simulink model "uz_mpc_prediction_state_machine"  (R2021a)
settings: Solver=FixedStepDiscrete  StartTime=0.0  StopTime=1/f*3  RelTol=1e-3
values from neighbouring files (symbols this model uses):
  A = 1.0    (= 1)    [uz_6ph_pu_vsd_voltages_init.m]    (also in uz_mpc_6ph_init.m; uz_mpc_6ph_state_machine_init.m)
  f = n_rpm/60.0*p    (= 250)    [uz_6ph_pu_vsd_voltages_init.m]    (also in uz_mpc_6ph_init.m; uz_mpc_6ph_state_machine_init.m)
  Ld_over_LB = Ld/LB    [uz_6ph_pu_vsd_voltages_init.m]    (also in uz_mpc_6ph_init.m; uz_mpc_6ph_state_machine_init.m)
  Lq_over_LB = Lq/LB    [uz_6ph_pu_vsd_voltages_init.m]    (also in uz_mpc_6ph_init.m; uz_mpc_6ph_state_machine_init.m)
  omega_m = n_rpm*pi/30    (= 314.159265359)    [uz_6ph_pu_vsd_voltages_init.m]    (also in uz_mpc_6ph_init.m; uz_mpc_6ph_state_machine_init.m)
  omegaB = nR*2*pi()/60*p    [uz_6ph_pu_vsd_voltages_init.m]    (also in uz_mpc_6ph_init.m; uz_mpc_6ph_state_machine_init.m)
  psi_pm_over_psiB = psi_pm/psiB    [uz_6ph_pu_vsd_voltages_init.m]    (also in uz_mpc_6ph_init.m; uz_mpc_6ph_state_machine_init.m)
  Rs_over_ZB = Rs/ZB    [uz_6ph_pu_vsd_voltages_init.m]    (also in uz_mpc_6ph_init.m; uz_mpc_6ph_state_machine_init.m)
  t_ADC = 1/f_ADC    (= 1e-05)    [uz_6ph_pu_vsd_voltages_init.m]    (also in uz_mpc_6ph_init.m; uz_mpc_6ph_state_machine_init.m; uz_typeconv_init.m)
  t_clock = 1/f_clock    (= 1e-08)    [uz_6ph_pu_vsd_voltages_init.m]    (also in uz_mpc_6ph_init.m; uz_mpc_6ph_state_machine_init.m; uz_typeconv_init.m)
  Ts_times_ZB_over_Ld = Ts*ZB/Ld    [uz_6ph_pu_vsd_voltages_init.m]    (also in uz_mpc_6ph_init.m; uz_mpc_6ph_state_machine_init.m)
  Ts_times_ZB_over_Lq = Ts*ZB/Lq    [uz_6ph_pu_vsd_voltages_init.m]    (also in uz_mpc_6ph_init.m; uz_mpc_6ph_state_machine_init.m)
  Ts_times_ZB_over_Lx = Ts*ZB/Lx    [uz_6ph_pu_vsd_voltages_init.m]    (also in uz_mpc_6ph_init.m; uz_mpc_6ph_state_machine_init.m)
  Ts_times_ZB_over_Ly = Ts*ZB/Ly    [uz_6ph_pu_vsd_voltages_init.m]    (also in uz_mpc_6ph_init.m; uz_mpc_6ph_state_machine_init.m)
  v_dc = 565.0    (= 565)    [uz_6ph_pu_vsd_voltages_init.m]    (also in uz_mpc_6ph_init.m; uz_mpc_6ph_state_machine_init.m)
  VB = sqrt(2/3)*VR    [uz_6ph_pu_vsd_voltages_init.m]    (also in uz_mpc_6ph_init.m; uz_mpc_6ph_state_machine_init.m)
libraries: simulink x9, fl_lib x7, nesl_utility x7, ee_lib x2, hdlsllib x1
(part 1 of 2)
settings Model: DataTypeOverride=Off  Creator=micha  LastModifiedBy=micha
settings SolverCC: AlgebraicLoopSolver=TrustRegion
settings DataIOCC: LimitDataPoints=on  SaveOutput=off  SaveTime=off
settings OptimizationCC: BlockReduction=off  ConditionallyExecuteInputs=off  DefaultParameterBehavior=Inlined  LifeSpan=inf
settings DebuggingCC: AlgebraicLoopMsg=error  SingleTaskRateTransMsg=error  AllowSymbolicDim=off  StrictBusMsg=ErrorOnBusTreatedAsVector  SFUnexpectedBacktrackingDiag=warning  SFNoUnconditionalDefaultTransitionDiag=warning  SFExecutionAtInitializationDiag=none  SFMachineParentedDataDiag=warning  ArithmeticOperatorsInVariantConditions=warning
settings HardwareCC: ProdBitPerPointer=32  ProdBitPerSizeT=32  ProdBitPerPtrDiffT=32  ProdLargestAtomicFloat=None  ProdIntDivRoundTo=Undefined  ProdEndianess=Unspecified  ProdWordSize=32  ProdHWDeviceType=ASIC/FPGA->ASIC/FPGA  ProdEqTarget=off
settings SFSimCC: SimUseLocalCustomCode=off  CustomCodeUndefinedFunction=UseInterfaceOnly
settings RTWCC: RTWUseLocalCustomCode=off
settings CodeAppCC: StateflowObjectComments=on
settings GRTTargetCC: TargetLangStandard=C89/C90 (ANSI)
settings ConfigComp: CovScope=ReferencedModels  CovMetricSettings=dw  CovSaveCumulativeToWorkspaceVar=on  CovSaveSingleToWorkspaceVar=on  CovExternalEMLEnable=off  CovSFcnEnable=off

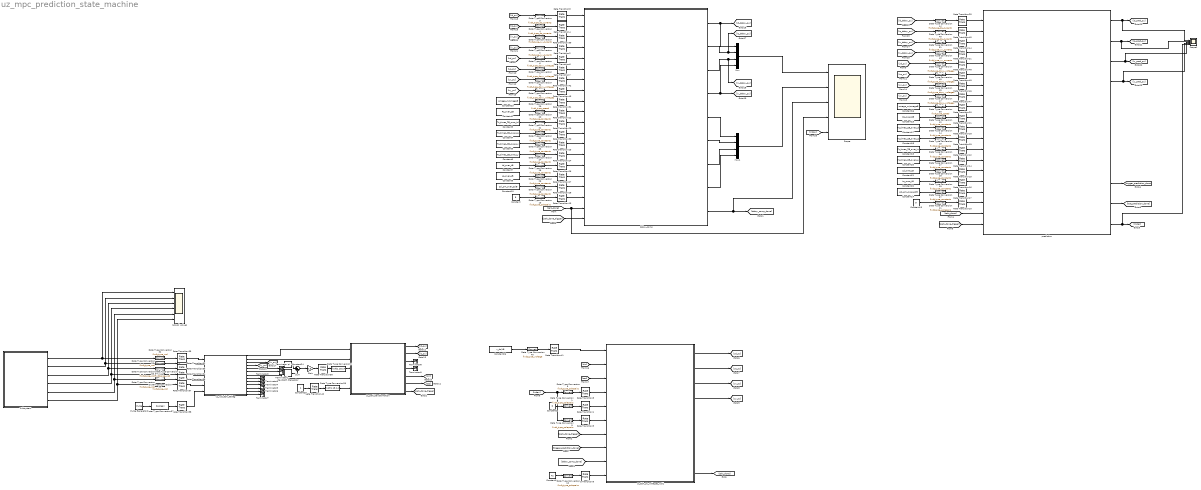
== system uz_mpc_prediction_state_machine ==
  Constant : Constant  Value=5
  Constant1 : Constant  Value=0
  Constant10 : Constant  Value=psi_pm_over_psiB
  Constant12 : Constant  Value=42
  Constant13 : Constant  Value=5
  Constant14 : Constant  Value=psi_pm_over_psiB
  Constant15 : Constant  Value=Rs_over_ZB
  Constant16 : Constant  Value=omega_m/omegaB
  Constant17 : Constant  Value=Ts_times_ZB_over_Ld
  Constant18 : Constant  Value=Ts_times_ZB_over_Lq
  Constant19 : Constant  Value=Ts_times_ZB_over_Lx
  Constant2 : Constant  Value=Rs_over_ZB
  Constant20 : Constant  Value=Ts_times_ZB_over_Ly
  Constant21 : Constant  Value=Ld_over_LB
  Constant22 : Constant  Value=Lq_over_LB
  Constant23 : Constant  Value=omega_m/omegaB
  Constant24 : Constant  Value=2*pi
  Constant25 : Constant
  Constant26 : Constant  Value=v_dc/VB
  Constant3 : Constant  Value=Ts_times_ZB_over_Ld
  Constant4 : Constant  Value=Ts_times_ZB_over_Lq
  Constant5 : Constant  Value=Ts_times_ZB_over_Lx
  Constant6 : Constant  Value=Ts_times_ZB_over_Ly
  Constant7 : Constant  Value=Ld_over_LB
  Constant8 : Constant  Value=Lq_over_LB
  Data Type Conversion{,2,31,43} (4 alike) : DataTypeConversion  OutDataTypeStr=fixdt_type_xy_currents
  Data Type Conversion{1,5,8,10..11,13} (6 alike) : DataTypeConversion  OutDataTypeStr=fixdt_type_polepairs
  Data Type Conversion{12,14..28} (16 alike) : DataTypeConversion  OutDataTypeStr=fixdt_type_constants
  Data Type Conversion29 : DataTypeConversion  OutDataTypeStr=fixdt_type_speed
  Data Type Conversion{3..4,44..45} (4 alike) : DataTypeConversion  OutDataTypeStr=fixdt_type_dq_currents
  Data Type Conversion30 : DataTypeConversion  OutDataTypeStr=fixdt_type_speed
  Data Type Conversion{32..36,38} (6 alike) : DataTypeConversion  OutDataTypeStr=fixdt_type_vsd
  Data Type Conversion37 : DataTypeConversion  OutDataTypeStr=boolean
  Data Type Conversion39 : DataTypeConversion  OutDataTypeStr=fixdt(1,18,14)
  Data Type Conversion40 : DataTypeConversion  OutDataTypeStr=fixdt_type_voltage
  Data Type Conversion{6..7,41..42,46..49} (8 alike) : DataTypeConversion  OutDataTypeStr=fixdt_type_dqxy_voltages
  Data Type Conversion9 : DataTypeConversion  OutDataTypeStr=fixdt(1,18,14)
  Gain : Gain  Gain=0.5
  Mux : Mux
  Mux1 : Mux
  Pulse Generator1 : DiscretePulseGenerator  PulseType=Time based  Period=t_ADC  PulseWidth=5
  Rate Transition{1,5,8..9} (4 alike) : RateTransition  InitialCondition=1  OutPortSampleTime=t_clock
  Rate Transition{2..4,6..7,10..49,58} (46 alike) : RateTransition  OutPortSampleTime=t_clock
  Sawtooth Generator : SignalGenerator  WaveForm=sawtooth  Amplitude=2*pi  Frequency=2*pi*f  Units=rad/sec
  Scope : Scope  NumInputPorts=5
  Scope1 : Scope  NumInputPorts=5
  Subsystem : Subsystem
  Sum : Sum  Inputs=|+-
  Terminator{,1..9} (10 alike) : Terminator
  delay_comp : Subsystem  TreatAsAtomicUnit=on
  natural values : Scope  NumInputPorts=6
  prediction : Subsystem  TreatAsAtomicUnit=on
  uz_6ph_pu_voltages_vsd1 : Subsystem  TreatAsAtomicUnit=on
  uz_park_transformation : Subsystem  TreatAsAtomicUnit=on
  uz_vsd_6ph_30deg : Subsystem  TreatAsAtomicUnit=on
  wires:
  Data Type Conversion24/1 -> Rate Transition24/1
  Constant8/1 -> Data Type Conversion26/1
  Rate Transition22/1 -> delay_comp/10(Rs_over_ZB_AXI)
  Data Type Conversion21/1 -> Rate Transition29/1
  Rate Transition29/1 -> delay_comp/11(Ts_times_ZB_over_Ld_AXI)
  Data Type Conversion26/1 -> Rate Transition27/1
  Constant6/1 -> Data Type Conversion24/1
  Rate Transition30/1 -> delay_comp/12(Ts_times_ZB_over_Lq_AXI)
  Rate Transition27/1 -> delay_comp/16(Lq_over_LB_AXI)
  Constant3/1 -> Data Type Conversion21/1
  Constant2/1 -> Data Type Conversion20/1
  Data Type Conversion25/1 -> Rate Transition26/1
  Data Type Conversion22/1 -> Rate Transition30/1
  Data Type Conversion23/1 -> Rate Transition23/1
  Rate Transition26/1 -> delay_comp/15(Ld_over_LB_AXI)
  Rate Transition24/1 -> delay_comp/14(Ts_times_ZB_over_Ly_AXI)
  Data Type Conversion20/1 -> Rate Transition22/1
  Rate Transition23/1 -> delay_comp/13(Ts_times_ZB_over_Lx_AXI)
  Constant5/1 -> Data Type Conversion23/1
  Constant4/1 -> Data Type Conversion22/1
  Constant7/1 -> Data Type Conversion25/1
  Data Type Conversion29/1 -> Rate Transition31/1
  Constant23/1 -> Data Type Conversion29/1
  Rate Transition31/1 -> delay_comp/9(omega_m_pu)
  Rate Transition2/1 -> delay_comp/4(iy_pu)
  Data Type Conversion3/1 -> Rate Transition3/1
  Rate Transition3/1 -> delay_comp/1(id_pu)
  Data Type Conversion4/1 -> Rate Transition4/1
  Data Type Conversion/1 -> Rate Transition39/1
  Data Type Conversion2/1 -> Rate Transition2/1
  Rate Transition4/1 -> delay_comp/2(iq_pu)
  Rate Transition39/1 -> delay_comp/3(ix_pu)
  Data Type Conversion6/1 -> Rate Transition6/1
  Rate Transition42/1 -> delay_comp/7(vx_pu)
  Data Type Conversion41/1 -> Rate Transition42/1
  Data Type Conversion7/1 -> Rate Transition7/1
  Data Type Conversion42/1 -> Rate Transition43/1
  Rate Transition6/1 -> delay_comp/5(vd_pu)
  Rate Transition7/1 -> delay_comp/6(vq_pu)
  Rate Transition43/1 -> delay_comp/8(vy_pu)
  uz_vsd_6ph_30deg/12(z1_AXI) -> Terminator6/1
  uz_park_transformation/4(y2_AXI) -> Terminator9/1
  uz_vsd_6ph_30deg/8(alpha_AXI) -> Terminator2/1
  uz_vsd_6ph_30deg/13(z2_AXI) -> Terminator7/1
  uz_park_transformation/3(y1_AXI) -> Terminator8/1
  uz_vsd_6ph_30deg/11(y_AXI) -> Terminator5/1
  Subsystem/1(output) -> natural values/1, Data Type Conversion32/1
  Data Type Conversion40/1 -> Rate Transition41/1
  Constant24/1 -> Sum/1
  uz_vsd_6ph_30deg/2(beta) -> uz_park_transformation/2(u2)
  Rate Transition35/1 -> uz_vsd_6ph_30deg/1(a1)
  Pulse Generator1/1 -> Data Type Conversion37/1
  Subsystem/2(output1) -> natural values/2, Data Type Conversion33/1
  uz_vsd_6ph_30deg/7(vsd_done) -> uz_park_transformation/4(trigger)
  Data Type Conversion39/1 -> uz_park_transformation/5(factor_angle_el_AXI)
  uz_vsd_6ph_30deg/1(alpha) -> uz_park_transformation/1(u1)
  Rate Transition41/1 -> uz_6ph_pu_voltages_vsd1/1(v_DC_pu)
  Rate Transition37/1 -> uz_vsd_6ph_30deg/6(c2)
  uz_vsd_6ph_30deg/10(x_AXI) -> Terminator4/1
  uz_vsd_6ph_30deg/6(z2) -> Terminator1/1
  uz_vsd_6ph_30deg/9(beta_AXI) -> Terminator3/1
  Subsystem/5(output4) -> Data Type Conversion36/1, natural values/5
  uz_6ph_pu_voltages_vsd1/9(calc_done) -> [calc_done]  "calc_done"
  Rate Transition33/1 -> uz_vsd_6ph_30deg/3(c1)
  uz_6ph_pu_voltages_vsd1/1(pu_ud) -> [ud_pu]
  Rate Transition38/1 -> Data Type Conversion9/1
  Data Type Conversion38/1 -> Rate Transition37/1
  Subsystem/4(output3) -> Data Type Conversion35/1, natural values/4
  Gain/1 -> Rate Transition38/1
  Rate Transition36/1 -> uz_vsd_6ph_30deg/5(b2)
  Sum/1 -> Gain/1
  Rate Transition58/1 -> uz_vsd_6ph_30deg/7(pu_conv_valid)
  Sawtooth Generator/1 -> Sum/2
  Constant25/1 -> Rate Transition40/1
  Rate Transition40/1 -> Data Type Conversion39/1
  Data Type Conversion34/1 -> Rate Transition33/1
  Subsystem/3(output2) -> Data Type Conversion34/1, natural values/3
  Rate Transition32/1 -> uz_vsd_6ph_30deg/2(b1)
  Subsystem/6(output5) -> natural values/6, Data Type Conversion38/1
  Data Type Conversion33/1 -> Rate Transition32/1
  Data Type Conversion32/1 -> Rate Transition35/1
  uz_vsd_6ph_30deg/5(z1) -> Terminator/1
  Data Type Conversion35/1 -> Rate Transition34/1
  Constant26/1 -> Data Type Conversion40/1
  Data Type Conversion36/1 -> Rate Transition36/1
  Data Type Conversion37/1 -> Rate Transition58/1
  Rate Transition34/1 -> uz_vsd_6ph_30deg/4(a2)
  Constant10/1 -> Data Type Conversion28/1
  Data Type Conversion28/1 -> Rate Transition28/1
  Rate Transition28/1 -> delay_comp/17(psi_pm_over_psiB_AXI)
  Constant/1 -> Data Type Conversion13/1
  Data Type Conversion13/1 -> Rate Transition13/1
  Rate Transition13/1 -> delay_comp/18(polepairs_AXI)
  delay_comp/1(id_delay_pu) -> [id_delay_pu], Mux/1
  delay_comp/2(iq_delay_pu) -> [iq_delay_pu], Mux/2
  delay_comp/3(ix_delay_pu) -> [ix_delay_pu], Mux/3
  delay_comp/4(iy_delay_pu) -> [iy_delay_pu], Mux/4
  Mux/1 -> Scope/1
  delay_comp/6(iq_delay_pu_AXI) -> Mux1/2
  delay_comp/8(iy_delay_pu_AXI) -> Mux1/4
  delay_comp/7(ix_delay_pu_AXI) -> Mux1/3
  delay_comp/5(id_delay_pu_AXI) -> Mux1/1
  Mux1/1 -> Scope/2
  delay_comp/9(calc_done) -> [delay_comp_done], Scope/3
  Rate Transition8/1 -> uz_6ph_pu_voltages_vsd1/4(index)
  Data Type Conversion5/1 -> Rate Transition8/1
  Rate Transition1/1 -> uz_6ph_pu_voltages_vsd1/5(index_select)
  Data Type Conversion1/1 -> Rate Transition1/1
  Constant1/1 -> Data Type Conversion1/1
  Rate Transition5/1 -> uz_6ph_pu_voltages_vsd1/6(index_AXI)
  Data Type Conversion8/1 -> Rate Transition5/1
  [index] -> Data Type Conversion8/1, Data Type Conversion5/1
  Data Type Conversion9/1 -> uz_park_transformation/3(angle_el)
  Data Type Conversion10/1 -> Rate Transition9/1
  Constant12/1 -> Data Type Conversion10/1
  Rate Transition9/1 -> uz_6ph_pu_voltages_vsd1/10(last_opt_index)
  [delay_comp_done] -> uz_6ph_pu_voltages_vsd1/9(trigger_delay_comp_done)
  uz_park_transformation/7(calc_done) -> [park_done_trigger]  "calc_done"
  [park_done_trigger] -> uz_6ph_pu_voltages_vsd1/7(trigger_adc)
  Data Type Conversion11/1 -> Rate Transition10/1
  Constant20/1 -> Data Type Conversion17/1
  Rate Transition10/1 -> prediction/18(polepairs_AXI)
  Constant13/1 -> Data Type Conversion11/1
  Constant14/1 -> Data Type Conversion27/1
  Constant22/1 -> Data Type Conversion19/1
  Data Type Conversion15/1 -> Rate Transition19/1
  Data Type Conversion19/1 -> Rate Transition16/1
  Constant18/1 -> Data Type Conversion15/1
  Rate Transition11/1 -> prediction/10(Rs_over_ZB_AXI)
  Rate Transition18/1 -> prediction/11(Ts_times_ZB_over_Ld_AXI)
  Data Type Conversion12/1 -> Rate Transition11/1
  Data Type Conversion16/1 -> Rate Transition12/1
  Constant16/1 -> Data Type Conversion30/1
  Rate Transition12/1 -> prediction/13(Ts_times_ZB_over_Lx_AXI)
  Rate Transition19/1 -> prediction/12(Ts_times_ZB_over_Lq_AXI)
  Data Type Conversion18/1 -> Rate Transition15/1
  Constant19/1 -> Data Type Conversion16/1
  Constant17/1 -> Data Type Conversion14/1
  Constant21/1 -> Data Type Conversion18/1
  Constant15/1 -> Data Type Conversion12/1
  Data Type Conversion27/1 -> Rate Transition17/1
  Rate Transition17/1 -> prediction/17(psi_pm_over_psiB_AXI)
  Rate Transition16/1 -> prediction/16(Lq_over_LB_AXI)
  Data Type Conversion30/1 -> Rate Transition20/1
  Rate Transition20/1 -> prediction/9(omega_m_pu)
  Rate Transition15/1 -> prediction/15(Ld_over_LB_AXI)
  Data Type Conversion17/1 -> Rate Transition14/1
  Data Type Conversion14/1 -> Rate Transition18/1
  Rate Transition14/1 -> prediction/14(Ts_times_ZB_over_Ly_AXI)
  Data Type Conversion31/1 -> Rate Transition44/1
  Rate Transition48/1 -> prediction/5(vd_pu)
  Data Type Conversion46/1 -> Rate Transition46/1
  Data Type Conversion44/1 -> Rate Transition25/1
  Data Type Conversion49/1 -> Rate Transition49/1
  Rate Transition25/1 -> prediction/1(id_pu)
  Rate Transition46/1 -> prediction/7(vx_pu)
  Data Type Conversion47/1 -> Rate Transition47/1
  Rate Transition47/1 -> prediction/8(vy_pu)
  Data Type Conversion43/1 -> Rate Transition21/1
  Rate Transition21/1 -> prediction/4(iy_pu)
  Data Type Conversion48/1 -> Rate Transition48/1
  Rate Transition44/1 -> prediction/3(ix_pu)
  Rate Transition45/1 -> prediction/2(iq_pu)
  Data Type Conversion45/1 -> Rate Transition45/1
  Rate Transition49/1 -> prediction/6(vq_pu)
  uz_6ph_pu_voltages_vsd1/2(pu_uq) -> [uq_pu]
  prediction/11(index) -> Scope1/5, [index]
  prediction/9(calc_done) -> [trigger_prediction_done]
  [trigger_prediction_done] -> uz_6ph_pu_voltages_vsd1/8(trigger_prediction_done)
  prediction/10(last_prediciton_done) -> [last_prediction_done]
  [calc_done] -> Scope/4, delay_comp/19(trigger_voltages_done)
  [park_done_trigger] -> delay_comp/20(adc_trigger)
  [calc_done] -> prediction/19(trigger_voltages_done)
  [park_done_trigger] -> prediction/20(adc_trigger)
  [ud_pu] -> Data Type Conversion6/1
  [ud_pu] -> Data Type Conversion48/1
  [uq_pu] -> Data Type Conversion7/1
  [uq_pu] -> Data Type Conversion49/1
  uz_6ph_pu_voltages_vsd1/3(pu_ux) -> [ux_pu]
  uz_6ph_pu_voltages_vsd1/4(pu_uy) -> [uy_pu]
  [uy_pu] -> Data Type Conversion42/1
  [ux_pu] -> Data Type Conversion41/1
  [ux_pu] -> Data Type Conversion46/1
  [uy_pu] -> Data Type Conversion47/1
  uz_park_transformation/5(sin) -> [sin]
  uz_park_transformation/6(cos) -> [cos]
  [cos] -> uz_6ph_pu_voltages_vsd1/3(cos_angle)
  [sin] -> uz_6ph_pu_voltages_vsd1/2(sin_angle)
  uz_park_transformation/1(y1) -> [id_pu]
  uz_park_transformation/2(y2) -> [iq_pu]
  [id_pu] -> Data Type Conversion3/1
  [iq_pu] -> Data Type Conversion4/1
  uz_vsd_6ph_30deg/4(y1) -> [iy_pu]
  uz_vsd_6ph_30deg/3(x1) -> [ix_pu]
  [iy_pu] -> Data Type Conversion2/1
  [ix_pu] -> Data Type Conversion/1
  [iy_delay_pu] -> Data Type Conversion43/1
  [ix_delay_pu] -> Data Type Conversion31/1
  [iq_delay_pu] -> Data Type Conversion45/1
  [id_delay_pu] -> Data Type Conversion44/1
  [index] -> Scope/5
  prediction/1(id_pred_pu) -> Scope1/1, [id_pred_pu]
  prediction/2(iq_pred_pu) -> Scope1/2, [iq_pred_pu]
  prediction/3(ix_pred_pu) -> Scope1/3, [ix_pred_pu]
  prediction/4(iy_pred_pu) -> Scope1/4, [iy_pred_pu]

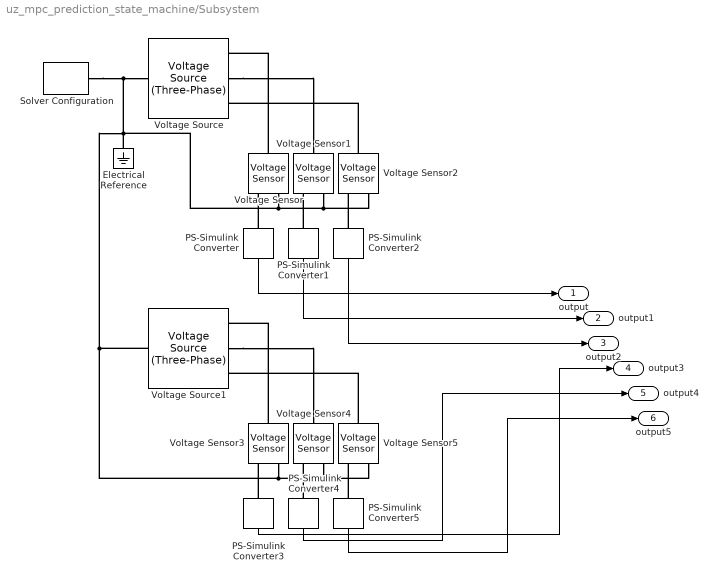
== system uz_mpc_prediction_state_machine/Subsystem ==
  Electrical Reference : fl_lib/Electrical/Electrical Elements/Electrical Reference
  PS-Simulink Converter{,1..5} (6 alike) : nesl_utility/PS-Simulink Converter  PhysicalDomain=network_engine_domain  SubClassName=ps_output  LeftPortType=input  RightPortType=output  PseudoPeriodic=off  Frequencies=[]  Unit=1  AffineConversion=off
  Solver Configuration : nesl_utility/Solver Configuration  PhysicalDomain=network_engine_domain  SubClassName=solver  LeftPortType=input  RightPortType=generic  Tones=[]  Harmonics=[]  SimulateNoise=off  Profile=off  UseLocalSampling=off  EnableSwitchedLinearOptims=on  FrequencyDomain=off  UseCCode=off  RelTol=0.001  AbsTol=1e-06  MinStep=1e-09  ToWorkspace=off  RevertToSquareIcSolve=off  NumHomotopyIterations=100  PhasorMode=off  PhasorModeNumHarmonics=1  DoDC=off  ResidualTolerance=1e-09  UseLocalSolver=on  LocalSolverChoice=NE_BACKWARD_EULER_ADVANCER  LocalSolverSampleTime=1e-6  DoFixedCost=on  MaxNonlinIter=3  MaxModeIter=2  ComputeImpulses=off  ImpulseIterations=2  LinearAlgebra=Sparse  EquationFormulation=NE_TIME_EF  DelaysMemoryBudget=1024  AutomaticFiltering=on  FilteringTimeConstant=0.001  PartitionStorageMethod=AS_NEEDED  PartitionMemoryBudget=1024  PartitionMethod=FAST
  Voltage Sensor{,1..5} (6 alike) : fl_lib/Electrical/Electrical Sensors/Voltage Sensor
  Voltage Source : ee_lib/Sources/Voltage Source (Three-Phase)  vline_rms=A*sqrt(3)/sqrt(2) V  shift=0 deg  freq=f Hz  impedance_option=1  SShortCircuit=1e6 V*A  XR=15  R=0.01 Ohm  L=3.97e-4 H  G_parasitic=0 1/Ohm  harmonic_option=1  harmonic_orders=Harmonic_Orders  harmonic_ratios=Harmonic_Amplitudes  I_specify=off  I_priority=None  I=[ 0 0 0 ] A  I_nominal_specify=off  I_nominal_unit=A  I_nominal_value=1
      settings: SourceProductBaseCode=PS  InternalSimscapePortConfiguration="{\"Bottom\":[],\"Left\":[{\"id\":\"n\",\"label\":\"n\",\"type\":\"foundation.electrical.electrical\"}],\"Right\":[{\"id\":\"a\",\"label\":\"a\",\"type\":\"foundation.electrical.electrical\"},{\"id\":\"b\",\"label\":\"b\",\"type\":\"foundation.electrical.electrical\"},{\"id\":\"c\",\"label\":\"c\",\"type\":\"foundation.electrical.electrical\"}],\"Top\":[]}"
  Voltage Source1 : ee_lib/Sources/Voltage Source (Three-Phase)  vline_rms=A*sqrt(3)/sqrt(2) V  shift=-30 deg  freq=f Hz  impedance_option=1  SShortCircuit=1e6 V*A  XR=15  R=0.01 Ohm  L=3.97e-4 H  G_parasitic=0 1/Ohm  harmonic_option=1  harmonic_orders=Harmonic_Orders  harmonic_ratios=Harmonic_Amplitudes  I_specify=off  I_priority=None  I=[ 0 0 0 ] A  I_nominal_specify=off  I_nominal_unit=A  I_nominal_value=1
      settings: SourceProductBaseCode=PS  InternalSimscapePortConfiguration="{\"Bottom\":[],\"Left\":[{\"id\":\"n\",\"label\":\"n\",\"type\":\"foundation.electrical.electrical\"}],\"Right\":[{\"id\":\"a\",\"label\":\"a\",\"type\":\"foundation.electrical.electrical\"},{\"id\":\"b\",\"label\":\"b\",\"type\":\"foundation.electrical.electrical\"},{\"id\":\"c\",\"label\":\"c\",\"type\":\"foundation.electrical.electrical\"}],\"Top\":[]}"
  output : Outport
  output1 : Outport  Port=2
  output2 : Outport  Port=3
  output3 : Outport  Port=4
  output4 : Outport  Port=5
  output5 : Outport  Port=6
  wires:
  PS-Simulink Converter/1 -> output/1
  PS-Simulink Converter3/1 -> output3/1
  PS-Simulink Converter4/1 -> output4/1
  PS-Simulink Converter1/1 -> output1/1
  PS-Simulink Converter5/1 -> output5/1
  PS-Simulink Converter2/1 -> output2/1
  connections:
  Voltage Sensor5/RConn2 -- Solver Configuration/RConn1 -- Voltage Source/LConn1 -- Voltage Sensor2/RConn2 -- Voltage Sensor1/RConn2 -- Voltage Sensor/RConn2 -- Electrical Reference/LConn1 -- Voltage Source1/LConn1 -- Voltage Sensor3/RConn2 -- Voltage Sensor4/RConn2
  PS-Simulink Converter5/LConn1 -- Voltage Sensor5/RConn1
  PS-Simulink Converter1/LConn1 -- Voltage Sensor1/RConn1
  Voltage Sensor3/LConn1 -- Voltage Source1/RConn1
  PS-Simulink Converter/LConn1 -- Voltage Sensor/RConn1
  Voltage Source1/RConn2 -- Voltage Sensor4/LConn1
  Voltage Sensor5/LConn1 -- Voltage Source1/RConn3
  PS-Simulink Converter4/LConn1 -- Voltage Sensor4/RConn1
  Voltage Sensor2/LConn1 -- Voltage Source/RConn3
  PS-Simulink Converter2/LConn1 -- Voltage Sensor2/RConn1
  PS-Simulink Converter3/LConn1 -- Voltage Sensor3/RConn1
  Voltage Sensor/LConn1 -- Voltage Source/RConn1
  Voltage Source/RConn2 -- Voltage Sensor1/LConn1

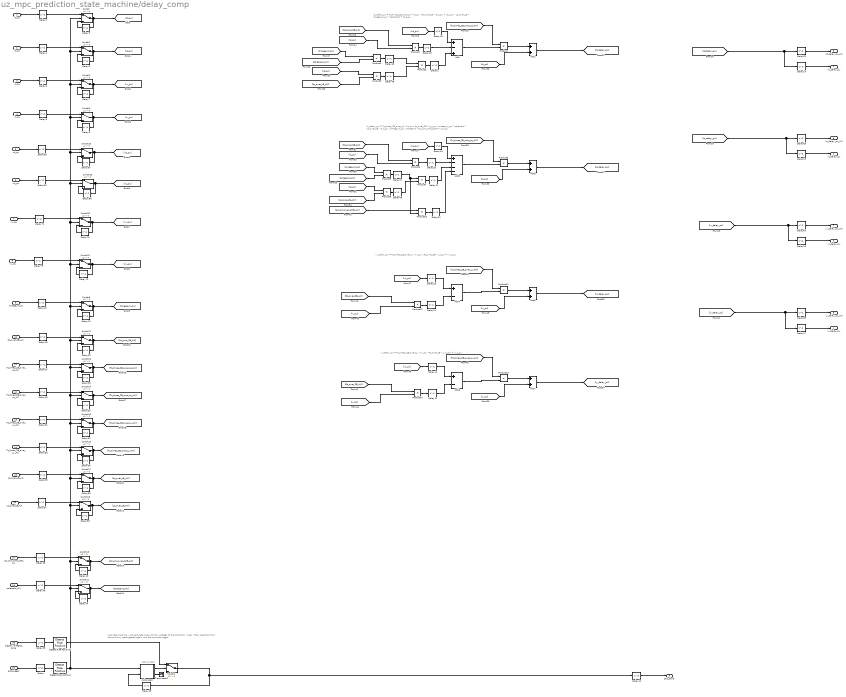
== system uz_mpc_prediction_state_machine/delay_comp ==
  note: mpc state machine - just calculate once with the voltages of the last optim. index. Then reset the S flip flop and only
      | get triggered again with the next adc trigger
  note: iy_delay_pu = Ts_times_ZB_over_Ly *(vy_pu - Rs_over_ZB * iy_k_pu) + iy_k_pu
  note: ix_delay_pu = Ts_times_ZB_over_Lx *(vx_pu - Rs_over_ZB* ix_k_pu) + ix_k_pu
  note: iq_delay_pu = Ts_times_ZB_over_Lq *(vq_pu - Rs_over_ZB * iq_k_pu - omega_m_pu * polepairs * Ld_over_LB * id_k_pu - omega_m_pu * polepairs * psi_pm_over_psiB) + iq_k_pu
  note: id_delay_pu = Ts_times_ZB_over_Ld *(vd_pu - Rs_over_ZB * id_k_pu + iq_k_pu * Lq_over_LB * omega_m_pu * polepairs) + id_k_pu
  note: Q=1 at start
  id_pu : Inport  OutDataTypeStr=fixdt_type_dq_currents
  iq_pu : Inport  Port=2  OutDataTypeStr=fixdt_type_dq_currents
  ix_pu : Inport  Port=3  OutDataTypeStr=fixdt_type_xy_currents
  iy_pu : Inport  Port=4  OutDataTypeStr=fixdt_type_xy_currents
  vd_pu : Inport  Port=5  OutDataTypeStr=fixdt_type_dqxy_voltages
  vq_pu : Inport  Port=6  OutDataTypeStr=fixdt_type_dqxy_voltages
  vx_pu : Inport  Port=7  OutDataTypeStr=fixdt_type_dqxy_voltages
  vy_pu : Inport  Port=8  OutDataTypeStr=fixdt_type_dqxy_voltages
  omega_m_pu : Inport  Port=9  OutDataTypeStr=fixdt_type_speed
  Rs_over_ZB_AXI : Inport  Port=10  OutDataTypeStr=fixdt_type_constants
  Ts_times_ZB_over_Ld_AXI : Inport  Port=11  OutDataTypeStr=fixdt_type_constants
  Ts_times_ZB_over_Lq_AXI : Inport  Port=12  OutDataTypeStr=fixdt_type_constants
  Ts_times_ZB_over_Lx_AXI : Inport  Port=13  OutDataTypeStr=fixdt_type_constants
  Ts_times_ZB_over_Ly_AXI : Inport  Port=14  OutDataTypeStr=fixdt_type_constants
  Ld_over_LB_AXI : Inport  Port=15  OutDataTypeStr=fixdt_type_constants
  Lq_over_LB_AXI : Inport  Port=16  OutDataTypeStr=fixdt_type_constants
  psi_pm_over_psiB_AXI : Inport  Port=17  OutDataTypeStr=fixdt_type_constants
  polepairs_AXI : Inport  Port=18  OutDataTypeStr=fixdt_type_polepairs
  trigger_voltages_done : Inport  Port=19
  adc_trigger : Inport  Port=20
  Add : Sum  Inputs=+-+  AccumDataTypeStr=fixdt(1,27,16)
  Add{1,3,5,7} (4 alike) : Sum  AccumDataTypeStr=fixdt(1,27,24)
  Add2 : Sum  Inputs=+---  AccumDataTypeStr=fixdt(1,27,16)
  Add4 : Sum  Inputs=+-  AccumDataTypeStr=fixdt(1,27,16)
  Add6 : Sum  Inputs=+-  AccumDataTypeStr=fixdt(1,27,16)
  Delay{,2,4,6,8,11..12,14..17,25,27,29,31,33,35,37,39,43,50,59..60,62..65,71,73} (29 alike) : Delay
  Delay{1,3,5,7,9..10,13,18..24,26,28,30,32,34,36,38,40..42,44..49,57..58,70,72} (34 alike) : Delay  DelayLength=1
  Detect Rise Positive : simulink/Logic and Bit Operations/Detect Rise Positive  vinit=0  OutDataTypeStr=boolean
  Detect Rise Positive1 : simulink/Logic and Bit Operations/Detect Rise Positive  vinit=0  OutDataTypeStr=boolean
  Product{,1..2,4..7,9..14} (13 alike) : Product  OutDataTypeStr=fixdt(1,18,15)
  Product3 : Product  OutDataTypeStr=fixdt(1,27,16)
  Product8 : Product  OutDataTypeStr=fixdt(1,27,16)
  Subsystem : Subsystem
  Switch : Switch  Criteria=u2 > Threshold  OutDataTypeStr=fixdt_type_dq_currents
  Switch1 : Switch  Criteria=u2 > Threshold  OutDataTypeStr=fixdt_type_dq_currents
  Switch{12..19} (8 alike) : Switch  Criteria=u2 > Threshold  OutDataTypeStr=fixdt_type_constants
  Switch2 : Switch  Criteria=u2 > Threshold  OutDataTypeStr=fixdt_type_xy_currents
  Switch21 : Switch  Criteria=u2 > Threshold  OutDataTypeStr=fixdt_type_polepairs
  Switch{28..31} (4 alike) : Switch  Criteria=u2 > Threshold  OutDataTypeStr=fixdt_type_dqxy_voltages
  Switch3 : Switch  Criteria=u2 > Threshold  OutDataTypeStr=fixdt_type_xy_currents
  Switch4 : Switch  Criteria=u2 > Threshold
  Switch5 : Switch  Criteria=u2 > Threshold  OutDataTypeStr=fixdt_type_speed
  Terminator2 : Terminator
  id_delay_pu : Outport
  iq_delay_pu : Outport  Port=2
  ix_delay_pu : Outport  Port=3
  iy_delay_pu : Outport  Port=4
  id_delay_pu_AXI : Outport  Port=5
  iq_delay_pu_AXI : Outport  Port=6
  ix_delay_pu_AXI : Outport  Port=7
  iy_delay_pu_AXI : Outport  Port=8
  calc_done : Outport  Port=9
  wires:
  Add5/1 -> [ix_delay_pu]
  Switch12/1 -> [Rs_over_ZB_AXI], Delay26/1
  Add3/1 -> [iq_delay_pu]
  Add1/1 -> [id_delay_pu]
  Add7/1 -> [iy_delay_pu]
  Delay5/1 -> Switch1/3
  Delay25/1 -> Switch12/1
  Delay59/1 -> Switch28/1
  Delay33/1 -> Switch16/1
  vx_pu/1 -> Delay71/1
  vd_pu/1 -> Delay59/1
  Switch15/1 -> [Ts_times_ZB_over_Lx_AXI], Delay32/1
  Ld_over_LB_AXI/1 -> Delay35/1
  Delay2/1 -> Switch/1
  Switch16/1 -> Delay34/1, [Ts_times_ZB_over_Ly_AXI]
  ix_pu/1 -> Delay6/1
  Delay38/1 -> Switch18/3
  Switch17/1 -> Delay36/1, [Ld_over_LB_AXI]
  Delay9/1 -> Switch3/3
  Switch13/1 -> [Ts_times_ZB_over_Ld_AXI], Delay28/1
  Delay/1 -> Detect Rise Positive/1
  Delay34/1 -> Switch16/3
  Delay44/1 -> Switch21/3
  Delay29/1 -> Switch14/1
  Delay8/1 -> Switch3/1
  Switch29/1 -> [vq_pu], Delay58/1
  Switch3/1 -> [iy_pu], Delay9/1
  polepairs_AXI/1 -> Delay43/1
  Delay72/1 -> Switch31/3
  Delay43/1 -> Switch21/1
  Switch14/1 -> [Ts_times_ZB_over_Lq_AXI], Delay30/1
  Delay28/1 -> Switch13/3
  psi_pm_over_psiB_AXI/1 -> Delay39/1
  Delay58/1 -> Switch29/3
  id_pu/1 -> Delay2/1
  Switch21/1 -> [polepairs_AXI], Delay44/1
  Switch/1 -> [id_pu], Delay3/1
  Delay35/1 -> Switch17/1
  Delay31/1 -> Switch15/1
  Switch28/1 -> [vd_pu], Delay57/1
  Ts_times_ZB_over_Ly_AXI/1 -> Delay33/1
  Delay7/1 -> Switch2/3
  Delay37/1 -> Switch18/1
  Delay4/1 -> Switch1/1
  Switch2/1 -> [ix_pu], Delay7/1
  Delay12/1 -> Switch5/1
  Delay73/1 -> Switch31/1
  Switch31/1 -> Delay72/1, [vy_pu]
  omega_m_pu/1 -> Delay12/1
  Delay6/1 -> Switch2/1
  Delay27/1 -> Switch13/1
  vq_pu/1 -> Delay60/1
  Switch5/1 -> [omega_m_pu], Delay13/1
  Lq_over_LB_AXI/1 -> Delay37/1
  iq_pu/1 -> Delay4/1
  iy_pu/1 -> Delay8/1
  vy_pu/1 -> Delay73/1
  Delay70/1 -> Switch30/3
  Delay60/1 -> Switch29/1
  Switch30/1 -> Delay70/1, [vx_pu]
  Ts_times_ZB_over_Lq_AXI/1 -> Delay29/1
  Delay3/1 -> Switch/3
  Switch18/1 -> Delay38/1, [Lq_over_LB_AXI]
  Delay26/1 -> Switch12/3
  Switch19/1 -> [psi_pm_over_psiB_AXI], Delay40/1
  Ts_times_ZB_over_Lx_AXI/1 -> Delay31/1
  Delay71/1 -> Switch30/1
  Switch1/1 -> [iq_pu], Delay5/1
  Ts_times_ZB_over_Ld_AXI/1 -> Delay27/1
  Delay57/1 -> Switch28/3
  Rs_over_ZB_AXI/1 -> Delay25/1
  Delay39/1 -> Switch19/1
  adc_trigger/1 -> Delay/1
  Delay40/1 -> Switch19/3
  Delay13/1 -> Switch5/3
  Delay32/1 -> Switch15/3
  Delay36/1 -> Switch17/3
  Delay30/1 -> Switch14/3
  Delay11/1 -> calc_done/1
  [iy_delay_pu] -> Delay17/1, Delay65/1
  [iq_delay_pu] -> Delay15/1, Delay63/1
  [id_delay_pu] -> Delay14/1, Delay62/1
  Delay63/1 -> iq_delay_pu_AXI/1
  Delay65/1 -> iy_delay_pu_AXI/1
  Delay64/1 -> ix_delay_pu_AXI/1
  [ix_delay_pu] -> Delay16/1, Delay64/1
  Delay62/1 -> id_delay_pu_AXI/1
  Delay15/1 -> iq_delay_pu/1
  Delay14/1 -> id_delay_pu/1
  Delay16/1 -> ix_delay_pu/1
  Delay17/1 -> iy_delay_pu/1
  Add/1 -> Product/2
  [Ts_times_ZB_over_Ld_AXI] -> Product/1  "Ts_times_ZB_over_Ld"
  Product/1 -> Add1/1
  [id_pu] -> Add1/2  "id_k_pu"
  [Rs_over_ZB_AXI] -> Product1/1  "Rs_over_ZB"
  [id_pu] -> Product1/2  "id_k_pu"
  [iq_pu] -> Product3/1  "iq_k_pu"
  [Lq_over_LB_AXI] -> Product3/2  "Lq_over_LB"
  [omega_m_pu] -> Product4/1  "omega_m_pu"
  [polepairs_AXI] -> Product4/2  "polepairs"
  [Ts_times_ZB_over_Lq_AXI] -> Product5/1  "Ts_times_ZB_over_Lq"
  [iq_pu] -> Product6/2  "iq_k_pu"
  [Rs_over_ZB_AXI] -> Product6/1  "Rs_over_ZB"
  Add2/1 -> Product5/2
  [omega_m_pu] -> Product9/1  "omega_m_pu"
  [iq_pu] -> Add3/2  "iq_k_pu"
  [id_pu] -> Product8/1  "id_k_pu"
  [Ld_over_LB_AXI] -> Product8/2  "Ld_over_LB"
  [polepairs_AXI] -> Product9/2  "polepairs"
  Product5/1 -> Add3/1
  [psi_pm_over_psiB_AXI] -> Product10/1
  [Ts_times_ZB_over_Lx_AXI] -> Product11/1  "Ts_times_ZB_over_Lx"
  [ix_pu] -> Product12/2  "ix_k_pu"
  [Rs_over_ZB_AXI] -> Product12/1  "Rs_over_ZB"
  Add4/1 -> Product11/2
  [ix_pu] -> Add5/2  "ix_k_pu"
  Product11/1 -> Add5/1
  [Rs_over_ZB_AXI] -> Product14/1  "Rs_over_ZB"
  Add6/1 -> Product13/2
  [iy_pu] -> Add7/2  "iy_k_pu"
  [iy_pu] -> Product14/2  "iy_k_pu"
  [Ts_times_ZB_over_Ly_AXI] -> Product13/1  "Ts_times_ZB_over_Ly"
  Product13/1 -> Add7/1
  Product2/1 -> Delay1/1
  Product1/1 -> Delay10/1
  Delay10/1 -> Add/2
  Delay1/1 -> Add/3
  [vd_pu] -> Delay18/1  "vd_pu"
  Delay18/1 -> Add/1
  [vq_pu] -> Delay19/1  "vq_pu"
  Product7/1 -> Delay21/1
  Product10/1 -> Delay22/1
  Delay22/1 -> Add2/4
  Delay21/1 -> Add2/3
  Delay20/1 -> Add2/2
  Delay19/1 -> Add2/1
  Product6/1 -> Delay20/1
  [vx_pu] -> Delay23/1  "vx_pu"
  Delay23/1 -> Add4/1
  Product12/1 -> Delay24/1
  Delay24/1 -> Add4/2
  [vy_pu] -> Delay41/1  "vy_pu"
  Product14/1 -> Delay42/1
  Delay42/1 -> Add6/2
  Delay41/1 -> Add6/1
  Product4/1 -> Delay45/1
  Product3/1 -> Delay46/1
  Delay46/1 -> Product2/2
  Delay45/1 -> Product2/1
  Product9/1 -> Delay47/1
  Delay47/1 -> Product10/2, Product7/1
  Product8/1 -> Delay48/1
  Delay48/1 -> Product7/2
  Delay49/1 -> Subsystem/2(Reset)
  Switch4/1 -> Delay49/1, Delay11/1  "delay_comp_done"
  Detect Rise Positive1/1 -> Switch4/1  "delay_comp done"
  Subsystem/1(Q) -> Switch4/2  "Q"
  Subsystem/2(!Q) -> Terminator2/1
  trigger_voltages_done/1 -> Delay50/1
  Delay50/1 -> Detect Rise Positive1/1
  Detect Rise Positive/1 -> Subsystem/1(Set), Switch21/2, Switch19/2, Switch18/2, Switch17/2, Switch16/2, Switch15/2, Switch14/2, Switch13/2, Switch12/2, Switch5/2, Switch31/2, Switch30/2, Switch29/2, Switch28/2, Switch3/2, Switch2/2, Switch1/2, Switch/2

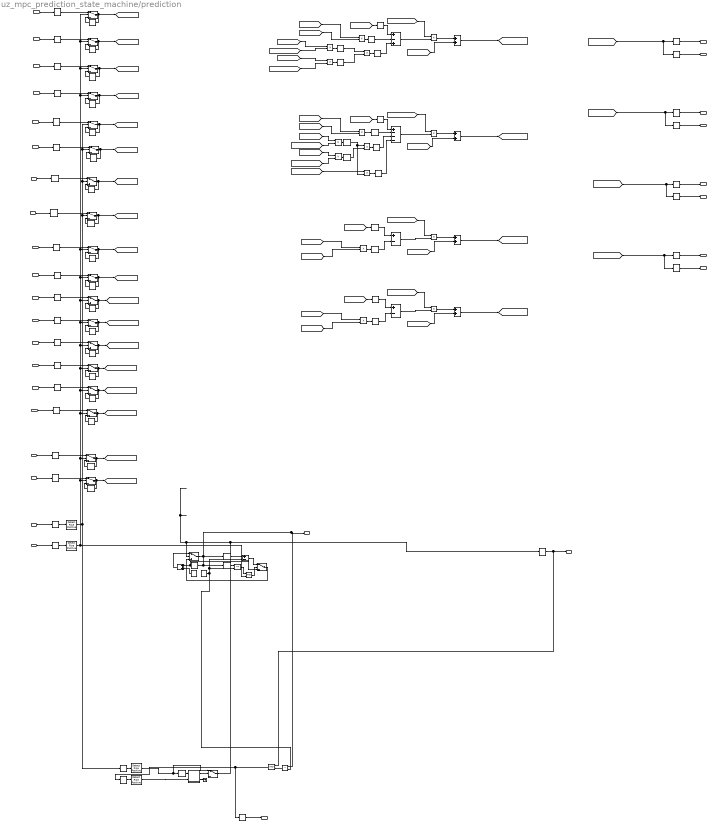
== system uz_mpc_prediction_state_machine/prediction ==
  note: voltages are triggered from voltage calculation ip every iteration
  note: iy_delay_pu = Ts_times_ZB_over_Ly *(vy_pu - Rs_over_ZB * iy_k_pu) + iy_k_pu
  note: ix_delay_pu = Ts_times_ZB_over_Lx *(vx_pu - Rs_over_ZB* ix_k_pu) + ix_k_pu
  note: iq_delay_pu = Ts_times_ZB_over_Lq *(vq_pu - Rs_over_ZB * iq_k_pu - omega_m_pu * polepairs * Ld_over_LB * id_k_pu - omega_m_pu * polepairs * psi_pm_over_psiB) + iq_k_pu
  note: id_delay_pu = Ts_times_ZB_over_Ld *(vd_pu - Rs_over_ZB * id_k_pu + iq_k_pu * Lq_over_LB * omega_m_pu * polepairs) + id_k_pu
  note: counter with adjustable reset
  note: mpc state machine
  id_pu : Inport  OutDataTypeStr=fixdt_type_dq_currents
  iq_pu : Inport  Port=2  OutDataTypeStr=fixdt_type_dq_currents
  ix_pu : Inport  Port=3  OutDataTypeStr=fixdt_type_xy_currents
  iy_pu : Inport  Port=4  OutDataTypeStr=fixdt_type_xy_currents
  vd_pu : Inport  Port=5  OutDataTypeStr=fixdt_type_dqxy_voltages
  vq_pu : Inport  Port=6  OutDataTypeStr=fixdt_type_dqxy_voltages
  vx_pu : Inport  Port=7  OutDataTypeStr=fixdt_type_dqxy_voltages
  vy_pu : Inport  Port=8  OutDataTypeStr=fixdt_type_dqxy_voltages
  omega_m_pu : Inport  Port=9  OutDataTypeStr=fixdt_type_speed
  Rs_over_ZB_AXI : Inport  Port=10  OutDataTypeStr=fixdt_type_constants
  Ts_times_ZB_over_Ld_AXI : Inport  Port=11  OutDataTypeStr=fixdt_type_constants
  Ts_times_ZB_over_Lq_AXI : Inport  Port=12  OutDataTypeStr=fixdt_type_constants
  Ts_times_ZB_over_Lx_AXI : Inport  Port=13  OutDataTypeStr=fixdt_type_constants
  Ts_times_ZB_over_Ly_AXI : Inport  Port=14  OutDataTypeStr=fixdt_type_constants
  Ld_over_LB_AXI : Inport  Port=15  OutDataTypeStr=fixdt_type_constants
  Lq_over_LB_AXI : Inport  Port=16  OutDataTypeStr=fixdt_type_constants
  psi_pm_over_psiB_AXI : Inport  Port=17  OutDataTypeStr=fixdt_type_constants
  polepairs_AXI : Inport  Port=18  OutDataTypeStr=fixdt_type_polepairs
  trigger_voltages_done : Inport  Port=19
  adc_trigger : Inport  Port=20
  Add : Sum  Inputs=+-+  AccumDataTypeStr=fixdt(1,27,16)
  Add{1,3,5,7} (4 alike) : Sum  AccumDataTypeStr=fixdt(1,27,24)
  Add2 : Sum  Inputs=+---  AccumDataTypeStr=fixdt(1,27,16)
  Add4 : Sum  Inputs=+-  AccumDataTypeStr=fixdt(1,27,16)
  Add6 : Sum  Inputs=+-  AccumDataTypeStr=fixdt(1,27,16)
  Add8 : Sum  AccumDataTypeStr=uint32
  Add9 : Sum  Inputs=+-  AccumDataTypeStr=uint32
  Constant : Constant  OutDataTypeStr=uint32  SampleTime=-1
  Constant1 : Constant  Value=63  OutDataTypeStr=uint32  SampleTime=-1
  Delay{,2,4,6,8,11..12,14..17,25,27,29,31,33,35,37,39,43,50,59..60,62..65,71,73} (29 alike) : Delay
  Delay{1,3,5,7,9..10,13,18..24,26,28,30,32,34,36,38,40..42,44..48,53..58,70,72} (37 alike) : Delay  DelayLength=1
  Delay49 : Delay  DelayLength=1  InitialCondition=1
  Delay51 : Delay  DelayLength=1  InitialCondition=1
  Delay52 : Delay  DelayLength=1  InitialCondition=1
  Detect Rise Positive{,1..3} (4 alike) : simulink/Logic and Bit Operations/Detect Rise Positive  vinit=0  OutDataTypeStr=boolean
  Logical Operator : Logic  AllPortsSameDT=off  OutDataTypeStr=boolean
  Logical Operator1 : Logic  AllPortsSameDT=off  OutDataTypeStr=boolean
  Product{,1..2,4..7,9..14} (13 alike) : Product  OutDataTypeStr=fixdt(1,18,15)
  Product3 : Product  OutDataTypeStr=fixdt(1,27,16)
  Product8 : Product  OutDataTypeStr=fixdt(1,27,16)
  Relational Operator : RelationalOperator  OutDataTypeStr=boolean  RndMeth=Simplest
  Relational Operator1 : RelationalOperator  Operator=>  OutDataTypeStr=boolean  RndMeth=Simplest
  Subsystem : Subsystem
  Switch : Switch  Criteria=u2 > Threshold  OutDataTypeStr=fixdt_type_dq_currents
  Switch1 : Switch  Criteria=u2 > Threshold  OutDataTypeStr=fixdt_type_dq_currents
  Switch{12..19} (8 alike) : Switch  Criteria=u2 > Threshold  OutDataTypeStr=fixdt_type_constants
  Switch2 : Switch  Criteria=u2 > Threshold  OutDataTypeStr=fixdt_type_xy_currents
  Switch21 : Switch  Criteria=u2 > Threshold  OutDataTypeStr=fixdt_type_polepairs
  Switch{28..31} (4 alike) : Switch  Criteria=u2 > Threshold  OutDataTypeStr=fixdt_type_dqxy_voltages
  Switch3 : Switch  Criteria=u2 > Threshold  OutDataTypeStr=fixdt_type_xy_currents
  Switch4 : Switch  Criteria=u2 > Threshold
  Switch5 : Switch  Criteria=u2 > Threshold  OutDataTypeStr=fixdt_type_speed
  Switch6 : Switch  Criteria=u2 > Threshold
  Switch7 : Switch  Criteria=u2 > Threshold
  Terminator1 : Terminator
  id_pred_pu : Outport
  iq_pred_pu : Outport  Port=2
  ix_pred_pu : Outport  Port=3
  iy_pred_pu : Outport  Port=4
  id_pred_pu_AXI : Outport  Port=5
  iq_pred_pu_AXI : Outport  Port=6
  ix_pred_pu_AXI : Outport  Port=7
  iy_pred_pu_AXI : Outport  Port=8
  calc_done : Outport  Port=9
  last_prediciton_done : Outport  Port=10  VectorParamsAs1DForOutWhenUnconnected=off
  index : Outport  Port=11  VectorParamsAs1DForOutWhenUnconnected=off
  wires:
  Add5/1 -> [ix_delay_pu]
  Switch12/1 -> [Rs_over_ZB_AXI], Delay26/1
  Add3/1 -> [iq_delay_pu]
  Add1/1 -> [id_delay_pu]
  Add7/1 -> [iy_delay_pu]
  Delay5/1 -> Switch1/3
  Delay25/1 -> Switch12/1
  Delay59/1 -> Switch28/1
  Delay33/1 -> Switch16/1
  vx_pu/1 -> Delay71/1
  vd_pu/1 -> Delay59/1
  Switch15/1 -> [Ts_times_ZB_over_Lx_AXI], Delay32/1
  Ld_over_LB_AXI/1 -> Delay35/1
  Delay2/1 -> Switch/1
  Switch16/1 -> Delay34/1, [Ts_times_ZB_over_Ly_AXI]
  ix_pu/1 -> Delay6/1
  Delay38/1 -> Switch18/3
  Switch17/1 -> Delay36/1, [Ld_over_LB_AXI]
  Delay9/1 -> Switch3/3
  Switch13/1 -> [Ts_times_ZB_over_Ld_AXI], Delay28/1
  Delay/1 -> Detect Rise Positive/1
  Delay34/1 -> Switch16/3
  Delay44/1 -> Switch21/3
  Delay29/1 -> Switch14/1
  Delay8/1 -> Switch3/1
  Switch29/1 -> [vq_pu], Delay58/1
  Switch3/1 -> [iy_pu], Delay9/1
  polepairs_AXI/1 -> Delay43/1
  Delay72/1 -> Switch31/3
  Delay43/1 -> Switch21/1
  Switch14/1 -> [Ts_times_ZB_over_Lq_AXI], Delay30/1
  Delay28/1 -> Switch13/3
  psi_pm_over_psiB_AXI/1 -> Delay39/1
  Delay58/1 -> Switch29/3
  id_pu/1 -> Delay2/1
  Switch21/1 -> [polepairs_AXI], Delay44/1
  Switch/1 -> [id_pu], Delay3/1
  Delay35/1 -> Switch17/1
  Delay31/1 -> Switch15/1
  Switch28/1 -> [vd_pu], Delay57/1
  Ts_times_ZB_over_Ly_AXI/1 -> Delay33/1
  Delay7/1 -> Switch2/3
  Delay37/1 -> Switch18/1
  Delay4/1 -> Switch1/1
  Switch2/1 -> [ix_pu], Delay7/1
  Delay12/1 -> Switch5/1
  Delay73/1 -> Switch31/1
  Switch31/1 -> Delay72/1, [vy_pu]
  omega_m_pu/1 -> Delay12/1
  Delay6/1 -> Switch2/1
  Delay27/1 -> Switch13/1
  vq_pu/1 -> Delay60/1
  Switch5/1 -> [omega_m_pu], Delay13/1
  Lq_over_LB_AXI/1 -> Delay37/1
  iq_pu/1 -> Delay4/1
  iy_pu/1 -> Delay8/1
  vy_pu/1 -> Delay73/1
  Delay70/1 -> Switch30/3
  Delay60/1 -> Switch29/1
  Switch30/1 -> Delay70/1, [vx_pu]
  Ts_times_ZB_over_Lq_AXI/1 -> Delay29/1
  Delay3/1 -> Switch/3
  Switch18/1 -> Delay38/1, [Lq_over_LB_AXI]
  Delay26/1 -> Switch12/3
  Switch19/1 -> [psi_pm_over_psiB_AXI], Delay40/1
  Ts_times_ZB_over_Lx_AXI/1 -> Delay31/1
  Delay71/1 -> Switch30/1
  Switch1/1 -> [iq_pu], Delay5/1
  Ts_times_ZB_over_Ld_AXI/1 -> Delay27/1
  Delay57/1 -> Switch28/3
  Rs_over_ZB_AXI/1 -> Delay25/1
  Delay39/1 -> Switch19/1
  adc_trigger/1 -> Delay/1
  Delay40/1 -> Switch19/3
  Delay13/1 -> Switch5/3
  Delay32/1 -> Switch15/3
  Delay36/1 -> Switch17/3
  Delay30/1 -> Switch14/3
  Delay11/1 -> Logical Operator1/1, calc_done/1
  [iy_delay_pu] -> Delay17/1, Delay65/1
  [iq_delay_pu] -> Delay15/1, Delay63/1
  [id_delay_pu] -> Delay14/1, Delay62/1
  Delay63/1 -> iq_pred_pu_AXI/1
  Delay65/1 -> iy_pred_pu_AXI/1
  Delay64/1 -> ix_pred_pu_AXI/1
  [ix_delay_pu] -> Delay16/1, Delay64/1
  Delay62/1 -> id_pred_pu_AXI/1
  Delay15/1 -> iq_pred_pu/1
  Delay14/1 -> id_pred_pu/1
  Delay16/1 -> ix_pred_pu/1
  Delay17/1 -> iy_pred_pu/1
  Add/1 -> Product/2
  [Ts_times_ZB_over_Ld_AXI] -> Product/1  "Ts_times_ZB_over_Ld"
  Product/1 -> Add1/1
  [id_pu] -> Add1/2  "id_k_pu"
  [Rs_over_ZB_AXI] -> Product1/1  "Rs_over_ZB"
  [id_pu] -> Product1/2  "id_k_pu"
  [iq_pu] -> Product3/1  "iq_k_pu"
  [Lq_over_LB_AXI] -> Product3/2  "Lq_over_LB"
  [omega_m_pu] -> Product4/1  "omega_m_pu"
  [polepairs_AXI] -> Product4/2  "polepairs"
  [Ts_times_ZB_over_Lq_AXI] -> Product5/1  "Ts_times_ZB_over_Lq"
  [iq_pu] -> Product6/2  "iq_k_pu"
  [Rs_over_ZB_AXI] -> Product6/1  "Rs_over_ZB"
  Add2/1 -> Product5/2
  [omega_m_pu] -> Product9/1  "omega_m_pu"
  [iq_pu] -> Add3/2  "iq_k_pu"
  [id_pu] -> Product8/1  "id_k_pu"
  [Ld_over_LB_AXI] -> Product8/2  "Ld_over_LB"
  [polepairs_AXI] -> Product9/2  "polepairs"
  Product5/1 -> Add3/1
  [psi_pm_over_psiB_AXI] -> Product10/1
  [Ts_times_ZB_over_Lx_AXI] -> Product11/1  "Ts_times_ZB_over_Lx"
  [ix_pu] -> Product12/2  "ix_k_pu"
  [Rs_over_ZB_AXI] -> Product12/1  "Rs_over_ZB"
  Add4/1 -> Product11/2
  [ix_pu] -> Add5/2  "ix_k_pu"
  Product11/1 -> Add5/1
  [Rs_over_ZB_AXI] -> Product14/1  "Rs_over_ZB"
  Add6/1 -> Product13/2
  [iy_pu] -> Add7/2  "iy_k_pu"
  [iy_pu] -> Product14/2  "iy_k_pu"
  [Ts_times_ZB_over_Ly_AXI] -> Product13/1  "Ts_times_ZB_over_Ly"
  Product13/1 -> Add7/1
  Product2/1 -> Delay1/1
  Product1/1 -> Delay10/1
  Delay10/1 -> Add/2
  Delay1/1 -> Add/3
  [vd_pu] -> Delay18/1  "vd_pu"
  Delay18/1 -> Add/1
  [vq_pu] -> Delay19/1  "vq_pu"
  Product7/1 -> Delay21/1
  Product10/1 -> Delay22/1
  Delay22/1 -> Add2/4
  Delay21/1 -> Add2/3
  Delay20/1 -> Add2/2
  Delay19/1 -> Add2/1
  Product6/1 -> Delay20/1
  [vx_pu] -> Delay23/1  "vx_pu"
  Delay23/1 -> Add4/1
  Product12/1 -> Delay24/1
  Delay24/1 -> Add4/2
  [vy_pu] -> Delay41/1  "vy_pu"
  Product14/1 -> Delay42/1
  Delay42/1 -> Add6/2
  Delay41/1 -> Add6/1
  Product4/1 -> Delay45/1
  Product3/1 -> Delay46/1
  Delay46/1 -> Product2/2
  Delay45/1 -> Product2/1
  Product9/1 -> Delay47/1
  Delay47/1 -> Product10/2, Product7/1
  Product8/1 -> Delay48/1
  Delay48/1 -> Product7/2
  Detect Rise Positive1/1 -> Delay53/1, Switch31/2, Switch30/2, Switch29/2, Switch28/2  "delay_comp done"
  trigger_voltages_done/1 -> Delay50/1
  Delay50/1 -> Detect Rise Positive1/1
  Add8/1 -> Switch4/1
  Relational Operator/1 -> Logical Operator/1
  Delay52/1 -> Add9/1
  Switch7/1 -> Switch4/2, Delay11/1  "trigger_predict"
  Detect Rise Positive/1 -> Switch21/2, Switch19/2, Switch18/2, Switch17/2, Switch16/2, Switch15/2, Switch14/2, Switch13/2, Switch12/2, Switch5/2, Switch3/2, Switch2/2, Switch1/2, Switch/2, Logical Operator/2
  Delay49/1 -> Switch6/3, Add8/1
  Add9/1 -> Switch6/1
  Constant/1 -> Add8/2
  Logical Operator/1 -> Switch6/2
  Delay51/1 -> Relational Operator/1
  Switch6/1 -> Switch4/3
  Switch4/1 -> Delay52/1, index/1, Relational Operator1/1, Delay49/1, Delay51/1  "predict done"
  Delay56/1 -> last_prediciton_done/1  "predict done"
  Detect Rise Positive3/1 -> Subsystem/2(Reset)
  Relational Operator1/1 -> Logical Operator1/2
  Delay54/1 -> Detect Rise Positive3/1
  Delay55/1 -> Subsystem/1(Set)
  Logical Operator1/1 -> Delay56/1, Delay54/1
  Subsystem/2(!Q) -> Terminator1/1
  Detect Rise Positive2/1 -> Switch7/1, Delay55/1
  Subsystem/1(Q) -> Switch7/2  "Q"
  Constant1/1 -> Relational Operator1/2, Add9/2, Relational Operator/2
  Delay53/1 -> Detect Rise Positive2/1

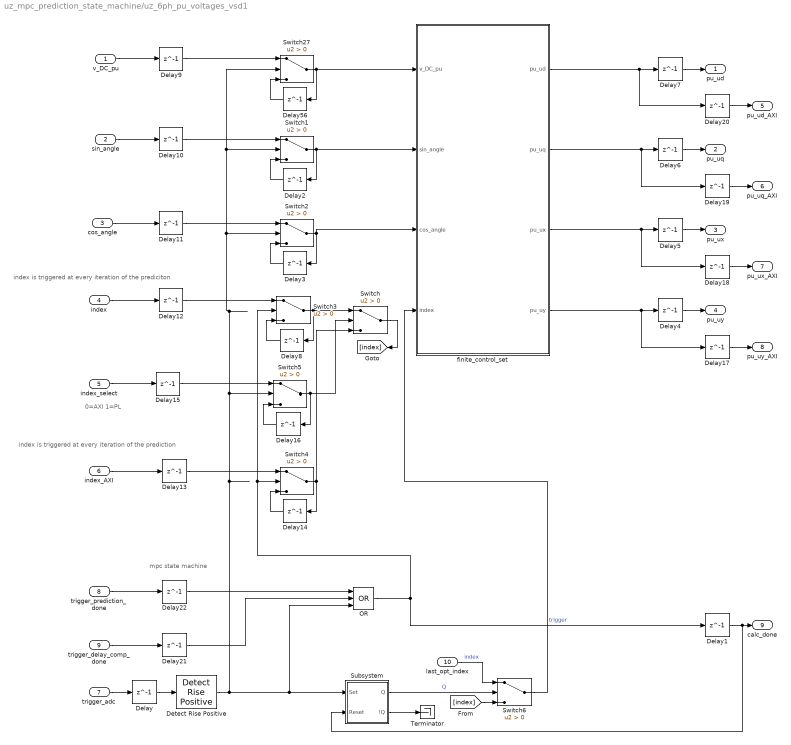
== system uz_mpc_prediction_state_machine/uz_6ph_pu_voltages_vsd1 ==
  note: index is triggered at every iteration of the prediction
  note: index is triggered at every iteration of the prediciton
  note: 0=AXI 1=PL
  note: mpc state machine
  v_DC_pu : Inport  OutDataTypeStr=fixdt_type_constants
  sin_angle : Inport  Port=2  OutDataTypeStr=fixdt_type_sin_cos
  cos_angle : Inport  Port=3  OutDataTypeStr=fixdt_type_sin_cos
  index : Inport  Port=4
  index_select : Inport  Port=5
  index_AXI : Inport  Port=6
  trigger_adc : Inport  Port=7
  trigger_prediction_done : Inport  Port=8
  trigger_delay_comp_done : Inport  Port=9
  last_opt_index : Inport  Port=10
  Delay{,1..7,9..13,15,17..22,56} (21 alike) : Delay  DelayLength=1
  Delay14 : Delay  DelayLength=1  InitialCondition=1
  Delay16 : Delay  DelayLength=1  InitialCondition=1
  Delay8 : Delay  DelayLength=1  InitialCondition=1
  Detect Rise Positive : simulink/Logic and Bit Operations/Detect Rise Positive  vinit=0  OutDataTypeStr=boolean
  OR : Logic  Operator=OR  Inputs=3  IconShape=distinctive  AllPortsSameDT=off  OutDataTypeStr=boolean
  Subsystem : Subsystem
  Switch : Switch  Criteria=u2 > Threshold
  Switch1 : Switch  Criteria=u2 > Threshold  OutDataTypeStr=fixdt_type_sin_cos
  Switch2 : Switch  Criteria=u2 > Threshold  OutDataTypeStr=fixdt_type_sin_cos
  Switch27 : Switch  Criteria=u2 > Threshold  OutDataTypeStr=fixdt_type_constants
  Switch3 : Switch  Criteria=u2 > Threshold  OutDataTypeStr=fixdt_type_polepairs
  Switch4 : Switch  Criteria=u2 > Threshold  OutDataTypeStr=fixdt_type_polepairs
  Switch5 : Switch  Criteria=u2 > Threshold  OutDataTypeStr=fixdt_type_polepairs
  Switch6 : Switch  Criteria=u2 > Threshold
  Terminator : Terminator
  finite_control_set : MATLAB Function  TreatAsAtomicUnit=on
  pu_ud : Outport
  pu_uq : Outport  Port=2
  pu_ux : Outport  Port=3
  pu_uy : Outport  Port=4
  pu_ud_AXI : Outport  Port=5
  pu_uq_AXI : Outport  Port=6
  pu_ux_AXI : Outport  Port=7
  pu_uy_AXI : Outport  Port=8
  calc_done : Outport  Port=9
  wires:
  finite_control_set/1(pu_ud) -> Delay20/1, Delay7/1
  finite_control_set/2(pu_uq) -> Delay19/1, Delay6/1
  finite_control_set/3(pu_ux) -> Delay18/1, Delay5/1
  finite_control_set/4(pu_uy) -> Delay17/1, Delay4/1
  trigger_adc/1 -> Delay/1
  Delay/1 -> Detect Rise Positive/1
  Delay56/1 -> Switch27/3
  v_DC_pu/1 -> Delay9/1
  Switch27/1 -> Delay56/1, finite_control_set/1(v_DC_pu)
  sin_angle/1 -> Delay10/1
  Delay2/1 -> Switch1/3
  Switch1/1 -> finite_control_set/2(sin_angle), Delay2/1
  cos_angle/1 -> Delay11/1
  Delay3/1 -> Switch2/3
  Switch2/1 -> finite_control_set/3(cos_angle), Delay3/1
  Delay4/1 -> pu_uy/1
  Delay5/1 -> pu_ux/1
  Delay6/1 -> pu_uq/1
  Delay7/1 -> pu_ud/1
  Switch3/1 -> Delay8/1, Switch/1
  index/1 -> Delay12/1
  Delay8/1 -> Switch3/3
  Delay9/1 -> Switch27/1
  Delay10/1 -> Switch1/1
  Delay11/1 -> Switch2/1
  Delay12/1 -> Switch3/1
  Delay14/1 -> Switch4/3
  index_AXI/1 -> Delay13/1
  Switch4/1 -> Switch/3, Delay14/1
  Delay13/1 -> Switch4/1
  Delay16/1 -> Switch5/3
  index_select/1 -> Delay15/1
  Switch5/1 -> Switch/2, Delay16/1
  Delay15/1 -> Switch5/1
  Delay17/1 -> pu_uy_AXI/1
  Delay19/1 -> pu_uq_AXI/1
  Delay20/1 -> pu_ud_AXI/1
  Delay18/1 -> pu_ux_AXI/1
  trigger_prediction_done/1 -> Delay22/1
  trigger_delay_comp_done/1 -> Delay21/1
  Delay21/1 -> OR/2
  OR/1 -> Switch3/2, Switch4/2, Delay1/1  "trigger"
  Delay22/1 -> OR/1
  Detect Rise Positive/1 -> Subsystem/1(Set), OR/3, Switch5/2, Switch2/2, Switch1/2, Switch27/2
  Subsystem/2(!Q) -> Terminator/1
  Delay1/1 -> Subsystem/2(Reset), calc_done/1
  Subsystem/1(Q) -> Switch6/2  "Q"
  last_opt_index/1 -> Switch6/1  "index"
  Switch/1 -> [index]
  [index] -> Switch6/3
  Switch6/1 -> finite_control_set/4(index)

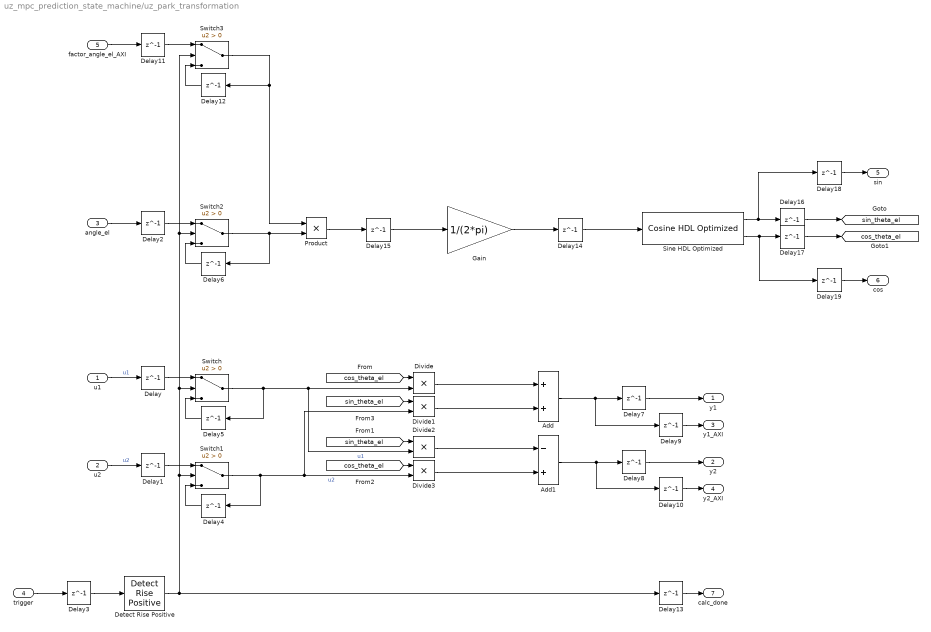
== system uz_mpc_prediction_state_machine/uz_park_transformation ==
  u1 : Inport
  u2 : Inport  Port=2
  angle_el : Inport  Port=3
  trigger : Inport  Port=4
  factor_angle_el_AXI : Inport  Port=5
  Add : Sum  OutDataTypeStr=fixdt(1,27,16)
  Add1 : Sum  Inputs=-+  OutDataTypeStr=fixdt(1,27,16)
  Delay{,1..19} (20 alike) : Delay  DelayLength=1
  Detect Rise Positive : simulink/Logic and Bit Operations/Detect Rise Positive  vinit=0  OutDataTypeStr=boolean
  Divide{,1..3} (4 alike) : Product  Inputs=**  OutDataTypeStr=fixdt(1,27,16)
  Gain : Gain  Gain=1/(2*pi)  OutDataTypeStr=fixdt(1,18,16)
  Product : Product  OutDataTypeStr=fixdt(1,18,14)
  Sine HDL Optimized : hdlsllib/Lookup Tables/Cosine HDL Optimized  OutputFormula=sin(2*pi*u) and cos(2*pi*u)  NumDataPoints=256  TableDataTypeStr=fixdt(0,17,16)  SimulateLUTROMDelay=off
      settings: SourceProductBaseCode=SL
  Switch{,1..3} (4 alike) : Switch  Criteria=u2 > Threshold
  y1 : Outport  VectorParamsAs1DForOutWhenUnconnected=off
  y2 : Outport  Port=2  VectorParamsAs1DForOutWhenUnconnected=off
  y1_AXI : Outport  Port=3  VectorParamsAs1DForOutWhenUnconnected=off
  y2_AXI : Outport  Port=4  VectorParamsAs1DForOutWhenUnconnected=off
  sin : Outport  Port=5  VectorParamsAs1DForOutWhenUnconnected=off
  cos : Outport  Port=6  VectorParamsAs1DForOutWhenUnconnected=off
  calc_done : Outport  Port=7  VectorParamsAs1DForOutWhenUnconnected=off
  tag scope: cos_theta_el=global, sin_theta_el=global
  wires:
  Switch1/1 -> Delay4/1, Divide1/2, Divide3/2  "u2"
  Divide2/1 -> Add1/1
  Divide3/1 -> Add1/2
  [cos_theta_el] -> Divide3/1
  Switch/1 -> Divide2/2, Divide/2, Delay5/1  "u1"
  [sin_theta_el] -> Divide2/1
  Divide1/1 -> Add/2
  [cos_theta_el] -> Divide/1
  [sin_theta_el] -> Divide1/1
  Add/1 -> Delay9/1, Delay7/1
  Add1/1 -> Delay10/1, Delay8/1
  Divide/1 -> Add/1
  angle_el/1 -> Delay2/1
  Sine HDL Optimized/2 -> Delay19/1, Delay17/1
  Sine HDL Optimized/1 -> Delay18/1, Delay16/1
  Gain/1 -> Delay14/1
  u1/1 -> Delay/1  "u1"
  u2/1 -> Delay1/1  "u2"
  Delay/1 -> Switch/1
  Delay1/1 -> Switch1/1
  Delay2/1 -> Switch2/1
  trigger/1 -> Delay3/1
  Delay4/1 -> Switch1/3
  Delay5/1 -> Switch/3
  Delay6/1 -> Switch2/3
  Delay7/1 -> y1/1
  Delay8/1 -> y2/1
  Delay9/1 -> y1_AXI/1
  Delay10/1 -> y2_AXI/1
  Switch2/1 -> Product/2, Delay6/1
  Switch3/1 -> Product/1, Delay12/1
  factor_angle_el_AXI/1 -> Delay11/1
  Detect Rise Positive/1 -> Delay13/1, Switch1/2, Switch/2, Switch3/2, Switch2/2
  Delay12/1 -> Switch3/3
  Delay11/1 -> Switch3/1
  Product/1 -> Delay15/1
  Delay3/1 -> Detect Rise Positive/1
  Delay13/1 -> calc_done/1
  Delay15/1 -> Gain/1
  Delay14/1 -> Sine HDL Optimized/1
  Delay16/1 -> [sin_theta_el]
  Delay17/1 -> [cos_theta_el]
  Delay18/1 -> sin/1
  Delay19/1 -> cos/1
